simulink model "Assignment_1"  (R2020b)
settings: Solver=VariableStepAuto  StartTime=0.0  StopTime=10.0  RelTol=1e-3
settings Model: Creator=Shantam Garg  LastModifiedBy=Shantam Garg

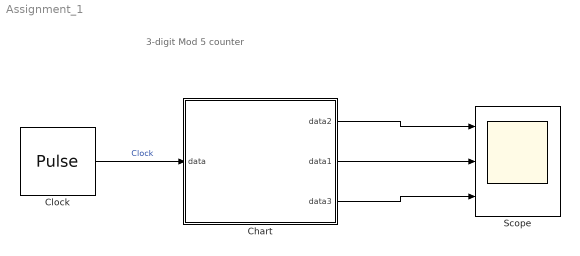
== system Assignment_1 ==
  note: 3-digit Mod 5 counter
  Chart : Stateflow chart  TreatAsAtomicUnit=on
  Clock : DiscretePulseGenerator  PulseType=Time based  Period=10  PulseWidth=5
  Scope : Scope  NumInputPorts=3
  wires:
  Clock/1 -> Chart/1(data)  "Clock"
  Chart/2(data1) -> Scope/2
  Chart/1(data2) -> Scope/1
  Chart/3(data3) -> Scope/3

== stateflow chart Assignment_1/Chart ==
  state State1
    en:
    a=0;
    b=0;
    c=0;
  state State2
    en:
    c=0;
    b=0;
    a=1;
  state State3
    en:
    c=0;
    b=1;
    a=0;
  state State4
    en:
    c=0;
    b=1;
    a=1;
  state State5
    en:
    c=1;
    b=0;
    a=0;
  (default) -> State1
  State5 -> State1
  State1 -> State2
  State2 -> State3
  State3 -> State4
  State4 -> State5
  data: data2 output; data input; data1 output; data3 output
